simulink model "l1outputfeedback"  (R2016a)
settings: Solver=ode1  StartTime=0.0  StopTime=100.0  FixedStep=1e-3  RelTol=1e-3
PreLoadFcn:
  | parameters
StartFcn:
  | parameters
values from neighbouring files (symbols this model uses):
  Gamma = 10    [configuration.m]    (also in parameters.m = 1)
  r = 3    [parameters.m]
  sigma = 2    [configuration.m]    (also in parameters.m = 1)
  tau = 1    [configuration.m]    (also in parameters.m = 0.1)
settings Model: Creator=Gabriel-Lenovo  LastModifiedBy=Gabriel-Lenovo

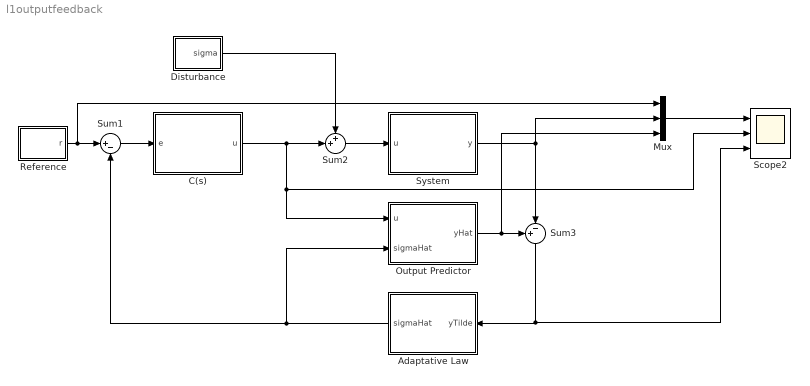
== system l1outputfeedback ==
  Adaptative Law : Subsystem
  C(s) : Subsystem
  Disturbance : Subsystem
  Mux : Mux  Inputs=3
  Output Predictor : Subsystem
  Reference : Subsystem
  Scope2 : Scope  NumInputPorts=3
  Sum1 : Sum  Inputs=|+-
  Sum2 : Sum  Inputs=++|
  Sum3 : Sum  Inputs=+-|
  System : Subsystem
  wires:
  Sum1/1 -> C(s)/1(e)
  Adaptative Law/1(sigmaHat) -> Sum1/2, Output Predictor/2(sigmaHat)
  Reference/1(r) -> Mux/1, Sum1/1
  Output Predictor/1(yHat) -> Mux/3, Sum3/1
  System/1(y) -> Mux/2, Sum3/2
  Disturbance/1(sigma) -> Sum2/1
  C(s)/1(u) -> Output Predictor/1("u "), Scope2/2, Sum2/2
  Sum2/1 -> System/1(u)
  Mux/1 -> Scope2/1
  Sum3/1 -> Scope2/3, Adaptative Law/1(yTilde)

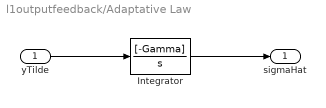
== system l1outputfeedback/Adaptative Law ==
  yTilde : Inport
  Integrator : TransferFcn  Numerator=[-Gamma]  Denominator=[1 0]
  sigmaHat : Outport
  wires:
  yTilde/1 -> Integrator/1
  Integrator/1 -> sigmaHat/1

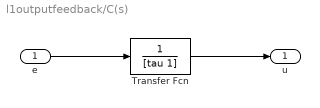
== system l1outputfeedback/C(s) ==
  e : Inport
  Transfer Fcn : TransferFcn  Denominator=[tau 1]
  u : Outport
  wires:
  e/1 -> Transfer Fcn/1
  Transfer Fcn/1 -> u/1

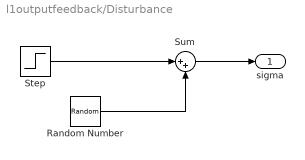
== system l1outputfeedback/Disturbance ==
  Random Number : RandomNumber  Variance=0
  Step : Step  Time=10  After=sigma*2  SampleTime=0
  Sum : Sum  Inputs=|++
  sigma : Outport
  wires:
  Step/1 -> Sum/1
  Random Number/1 -> Sum/2
  Sum/1 -> sigma/1

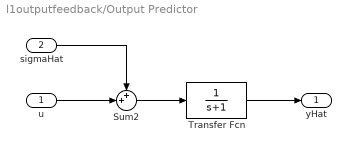
== system l1outputfeedback/Output Predictor ==
  "u " : Inport
  sigmaHat : Inport  Port=2
  Sum2 : Sum  Inputs=++|
  Transfer Fcn : TransferFcn  Denominator=[1 1]
  yHat : Outport
  wires:
  Transfer Fcn/1 -> yHat/1
  "u "/1 -> Sum2/2
  sigmaHat/1 -> Sum2/1
  Sum2/1 -> Transfer Fcn/1

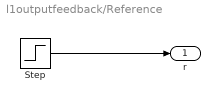
== system l1outputfeedback/Reference ==
  Step : Step  After=r  SampleTime=0
  r : Outport
  wires:
  Step/1 -> r/1

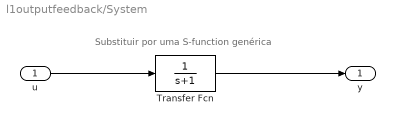
== system l1outputfeedback/System ==
  note: Substituir por uma S-function genérica
  u : Inport
  Transfer Fcn : TransferFcn  Denominator=[1 1]
  y : Outport
  wires:
  u/1 -> Transfer Fcn/1
  Transfer Fcn/1 -> y/1
